simulink model "Cv_1"  (R2024a)
settings: Solver=VariableStepAuto  StartTime=0.0  StopTime=5  MaxStep=1/2000  RelTol=1e-3
settings Model: Creator=221208  LastModifiedBy=Miloš Uhlíř
settings ModelReferenceCC: EnableRefExpFcnMdlSchedulingChecks=on
settings RTWCC: GPUComputeCapability=3.5

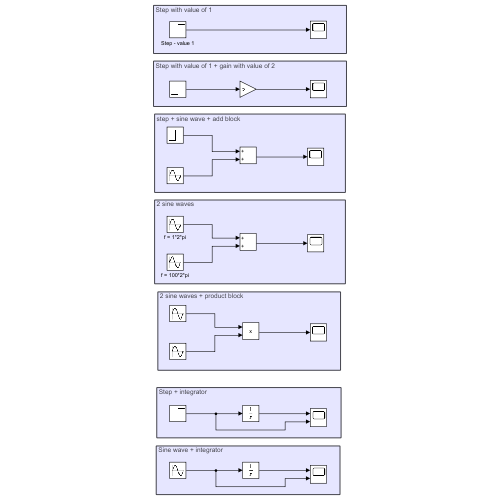
[thumbnail: Simulink's stored preview of the top-level diagram]
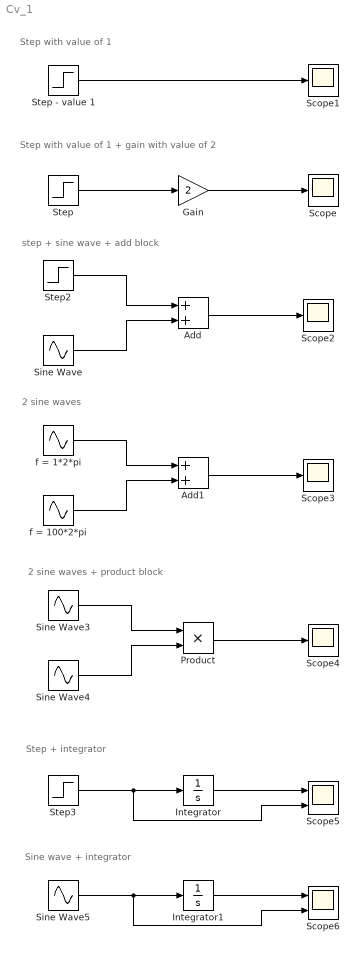
== system Cv_1 ==
  note: Sine wave + integrator
  note: Step + integrator
  note: 2 sine waves + product block
  note: 2 sine waves
  note: step + sine wave + add block
  note: Step with value of 1 + gain with value of 2
  note: Step with value of 1
  Add : Sum
  Add1 : Sum
  Gain : Gain  Gain=2
  Integrator : Integrator
  Integrator1 : Integrator
  Product : Product
  Scope{,1..4} (5 alike) : Scope
  Scope5 : Scope  NumInputPorts=2
  Scope6 : Scope  NumInputPorts=2
  Sine Wave : Sin  SampleTime=0
  Sine Wave3 : Sin  Frequency=1*2*pi  SampleTime=0
  Sine Wave4 : Sin  Frequency=100*2*pi  SampleTime=0
  Sine Wave5 : Sin  Frequency=2*2*pi  SampleTime=0
  Step : Step  SampleTime=0
  Step - value 1 : Step  SampleTime=0
  Step2 : Step  SampleTime=0
  Step3 : Step  SampleTime=0
  f = 1*2*pi : Sin  Frequency=1*2*pi  SampleTime=0
  f = 100*2*pi : Sin  Frequency=100*2*pi  SampleTime=0
  wires:
  Step/1 -> Gain/1
  Gain/1 -> Scope/1
  Step - value 1/1 -> Scope1/1
  Sine Wave/1 -> Add/2
  Step2/1 -> Add/1
  Add/1 -> Scope2/1
  f = 100*2*pi/1 -> Add1/2
  f = 1*2*pi/1 -> Add1/1
  Add1/1 -> Scope3/1
  Product/1 -> Scope4/1
  Sine Wave3/1 -> Product/1
  Sine Wave4/1 -> Product/2
  Step3/1 -> Scope5/2, Integrator/1
  Integrator/1 -> Scope5/1
  Sine Wave5/1 -> Scope6/2, Integrator1/1
  Integrator1/1 -> Scope6/1
